simulink model "rah"  (Simulink 2.09)
settings: Solver=ode15s  StartTime=0.0  StopTime=60  MaxStep=5  RelTol=1e-6  AbsTol=1e-6
values from neighbouring files (symbols this model uses):
  dar = 0.165    [kpahrah.m]
  drr = -0.000075*Vref^2 + 0.0095*Vref - 0.4606    (= -0.184975)    [kpahrah.m]
  Ki_2 = 0.25    [kpahrah.m]
  Kphi = 0.000975*Vref^2 - 0.108*Vref + 2.335625    (= -0.55)    [kpahrah.m]
  Kr = -4    [kpahrah.m]
  refvelocity = 55    [actrload.m]    (also in prahinit.m = 45)
undefined symbols (not defined in the file or in its folder): Aail, AM, Arud, Bail, Brud, Cail, Crud, Dail, Drud, GM1, uaero0, uprop0, xfix, xinco
settings Model: SaveTime=off  SaveOutput=off  ConsistencyChecking=off  RTWTemplateMakefile=grt_vc.tmf

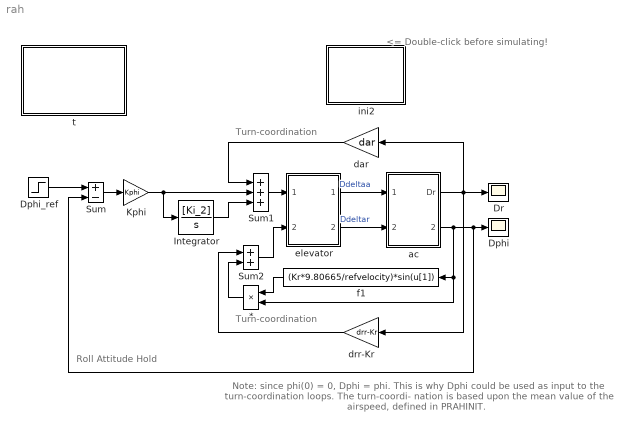
== system rah ==
  note: <= Double-click
      | before
      |   simulating!
  note: Note: since phi(0) = 0, Dphi = phi. This
      | is why Dphi could be used as input to the
      | turn-coordination loops. The turn-coordi-
      | nation is based upon the mean value of
      | the airspeed, defined in PRAHINIT.
  note: Roll Attitude Hold
  note: Turn-coordination
  note: Turn-coordination
  * : Product  Orientation=left  Inputs=2
  Dphi : Scope
      settings: TickLabels=on  TimeRange=60.000000  YMin=-0.300000  YMax=0.300000  SaveToWorkspace=off  SaveName=ScopeData
  Dphi_ref : Step  Time=0  Before=0  After=10*pi/180
  Dr : Scope
      settings: TickLabels=on  TimeRange=60.000000  YMin=-0.025000  YMax=0.025000  SaveToWorkspace=off  SaveName=ScopeData
  Integrator : TransferFcn  Numerator=[Ki_2]  Denominator=[1 0]
  Kphi : Gain  Gain=Kphi
  Sum : Sum  Inputs=+-
  Sum1 : Sum  Inputs=+++
  Sum2 : Sum  Inputs=++
  ac : Subsystem
      mask Display: disp('BEAVER\ndynamics')
  dar : Gain  Orientation=left  Gain=dar
  drr-Kr : Gain  Orientation=left  Gain=drr-Kr
  elevator : Subsystem
      mask Display: disp('Cable &\nactuator\ndynamics')
  f1 : Fcn  Orientation=left  Expr=(Kr*9.80665/refvelocity)*sin(u[1])
  ini2 : Subsystem
      settings: OpenFcn=prahinit
      mask Display: disp('Initialize\nmodel\n\nPRAHINIT')
  t : Subsystem
      mask Display: disp('RAH with\nturn-coordination\nwithout limiters.\nMarc Rauw,\nOctober 1997')
  wires:
  Dphi_ref/1 -> Sum/1
  Sum/1 -> Kphi/1
  elevator/1(Ddeltaa) -> ac/1(Ddelta_a)  "Ddeltaa"
  elevator/2(Ddeltar) -> ac/2(Ddelta_r)  "Ddeltar"
  Sum1/1 -> elevator/1(VDdeltaa)
  ac/1(Dr) -> Dr/1, dar/1, drr-Kr/1
  f1/1 -> */1
  Sum2/1 -> elevator/2(VDdeltar)
  */1 -> Sum2/2
  drr-Kr/1 -> Sum2/1
  ac/2(Dphi) -> f1/1, */2, Sum/2, Dphi/1
  Kphi/1 -> Sum1/2, Integrator/1
  Integrator/1 -> Sum1/3
  dar/1 -> Sum1/1

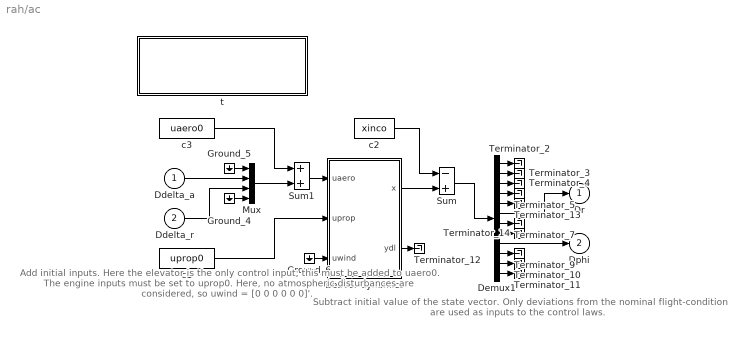
== system rah/ac ==
  note: Subtract initial value of  the state
      | vector. Only deviations from the
      | nominal flight-condition are used
      | as inputs to the control laws.
  note: Add initial inputs. Here the elevator
      | is the only control input; this must
      | be added to uaero0. The engine
      | inputs must be set to uprop0. Here,
      | no atmospheric disturbances are
      | considered, so uwind = [0 0 0 0 0 0]'.
  Ddelta_a : Inport  Port=1  PortWidth=-1  SampleTime=-1
  Ddelta_r : Inport  Port=2  PortWidth=-1  SampleTime=-1
  Beaver dynamics : Subsystem
  Demux1 : Demux  Outputs=12
  Ground_4 : Ground
  Ground_5 : Ground
  Ground_6 : Ground
  Mux : Mux  Inputs=4
  Sum : Sum  Inputs=-+
  Sum1 : Sum  Inputs=++
  Terminator_{2..5,7,9..14} (11 alike) : Terminator
  c1 : Constant  Value=uprop0
  c2 : Constant  Value=xinco
  c3 : Constant  Value=uaero0
  t : Subsystem
      mask Display: disp('Call subsystem-equivalent of the\nsystem BEAVER and convert\nI/O signals to small-deviations.\nMarc Rauw, October 1997')
  Dr : Outport  Port=1  InitialOutput=0
  Dphi : Outport  Port=2  InitialOutput=0
  wires:
  c3/1 -> Sum1/1
  c1/1 -> Beaver dynamics/2(uprop)
  c2/1 -> Sum/1
  Beaver dynamics/2(ydl) -> Terminator_12/1
  Beaver dynamics/1(x) -> Sum/2
  Demux1/1 -> Terminator_2/1
  Demux1/2 -> Terminator_3/1
  Demux1/3 -> Terminator_4/1
  Demux1/4 -> Terminator_5/1
  Demux1/7 -> Terminator_7/1
  Demux1/10 -> Terminator_9/1
  Demux1/11 -> Terminator_10/1
  Demux1/12 -> Terminator_11/1
  Sum/1 -> Demux1/1
  Sum1/1 -> Beaver dynamics/1(uaero)
  Mux/1 -> Sum1/2
  Ddelta_a/1 -> Mux/2
  Ground_5/1 -> Mux/1
  Ddelta_r/1 -> Mux/3
  Ground_4/1 -> Mux/4
  Ground_6/1 -> Beaver dynamics/3(uwind)
  Demux1/5 -> Terminator_13/1
  Demux1/8 -> Terminator_14/1
  Demux1/6 -> Dr/1
  Demux1/9 -> Dphi/1

== system rah/elevator ==
  note: Second inputs of Mux blocks take into account
      | influence of roll and yaw-rate upon aileron deflection
      | and rudder deflection, respectively (neglected here).
  VDdeltaa : Inport  Port=1  PortWidth=-1  SampleTime=-1
  VDdeltar : Inport  Port=2  PortWidth=-1  SampleTime=-1
  Ailerons actuator and cables : StateSpace  A=Aail  B=Bail  C=Cail  D=Dail  X0=0
  Ground_1 : Ground
  Ground_2 : Ground
  Mux : Mux  Inputs=2
  Mux1 : Mux  Inputs=2
  Rudder actuator and cables : StateSpace  A=Arud  B=Brud  C=Crud  D=Drud  X0=0
  t : Subsystem
      mask Display: disp('Dynamics of ailerons and\nrudder actuators and cables.\nMarc Rauw, October 1997')
  Ddeltaa : Outport  Port=1  InitialOutput=0
  Ddeltar : Outport  Port=2  InitialOutput=0
  wires:
  Ailerons actuator and cables/1 -> Ddeltaa/1
  VDdeltaa/1 -> Mux/1
  Mux/1 -> Ailerons actuator and cables/1
  Mux1/1 -> Rudder actuator and cables/1
  VDdeltar/1 -> Mux1/1
  Rudder actuator and cables/1 -> Ddeltar/1
  Ground_1/1 -> Mux/2
  Ground_2/1 -> Mux1/2

== system rah/ini2 ==

== system rah/t ==

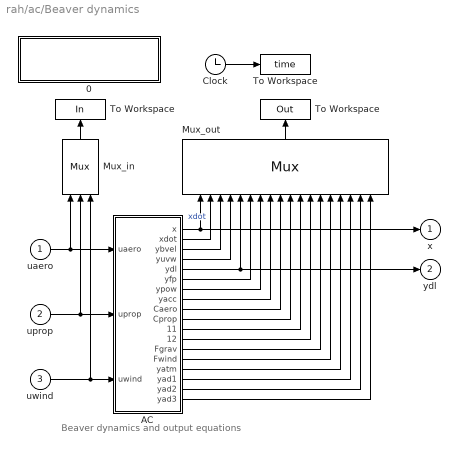
== system rah/ac/Beaver dynamics ==
  note: Beaver dynamics
      | and output equations
  uaero : Inport  Port=1  PortWidth=4  SampleTime=-1
  uprop : Inport  Port=2  PortWidth=2  SampleTime=-1
  uwind : Inport  Port=3  PortWidth=6  SampleTime=-1
  0 : Subsystem
      settings: OpenFcn=fdchelp level1
      mask Display: disp('Subsystem equivalent of\nthe S-function BEAVER\nM.O. Rauw, October 1997')
  AC : Subsystem
  Clock : Clock
  Mux_in : Mux  Orientation=up  Inputs=[4 2 6]
      settings: OpenFcn=fdchelp inputs
      mask Display: disp('Mux\nclick\n2x for\ninfo!')
  Mux_out : Mux  Orientation=up  Inputs=[12 12 3 3 3 4 2 6 6 6 6 6 3 3 5 3 3 3]
      settings: OpenFcn=fdchelp outputs
      mask Display: disp('Mux\n\nDouble-click for info!')
  To Workspace : ToWorkspace  VariableName=Out  SampleTime=0
      settings: Orientation=up  Buffer=5000
  "To Workspace " : ToWorkspace  VariableName=In  SampleTime=0
      settings: Orientation=up  Buffer=5000
  "To Workspace  " : ToWorkspace  VariableName=time  SampleTime=0
      settings: Buffer=5000
  x : Outport  Port=1  InitialOutput=0
  ydl : Outport  Port=2  InitialOutput=0
  wires:
  AC/7(ypow) -> Mux_out/7
  Mux_in/1 -> "To Workspace "/1
  Mux_out/1 -> To Workspace/1
  Clock/1 -> "To Workspace  "/1
  AC/15(yatm) -> Mux_out/15
  AC/14(Fwind) -> Mux_out/14
  AC/13(Fgrav) -> Mux_out/13
  AC/12(FMprop) -> Mux_out/12
  AC/11(FMaero) -> Mux_out/11
  AC/10(Cprop) -> Mux_out/10
  AC/9(Caero) -> Mux_out/9
  AC/8(yacc) -> Mux_out/8
  AC/6(yfp) -> Mux_out/6
  AC/5(ydl) -> ydl/1, Mux_out/5
  AC/16(yad1) -> Mux_out/16
  AC/3(ybvel) -> Mux_out/3
  AC/1(x) -> Mux_out/1, x/1
  AC/4(yuvw) -> Mux_out/4
  AC/17(yad2) -> Mux_out/17
  AC/18(yad3) -> Mux_out/18
  uwind/1 -> AC/3(" uwind"), Mux_in/3
  uprop/1 -> AC/2(uprop), Mux_in/2
  uaero/1 -> AC/1(uaero), Mux_in/1
  AC/2(xdot) -> Mux_out/2  "xdot"

== system rah/ac/t ==

== system rah/elevator/t ==

== system rah/ac/Beaver dynamics/0 ==

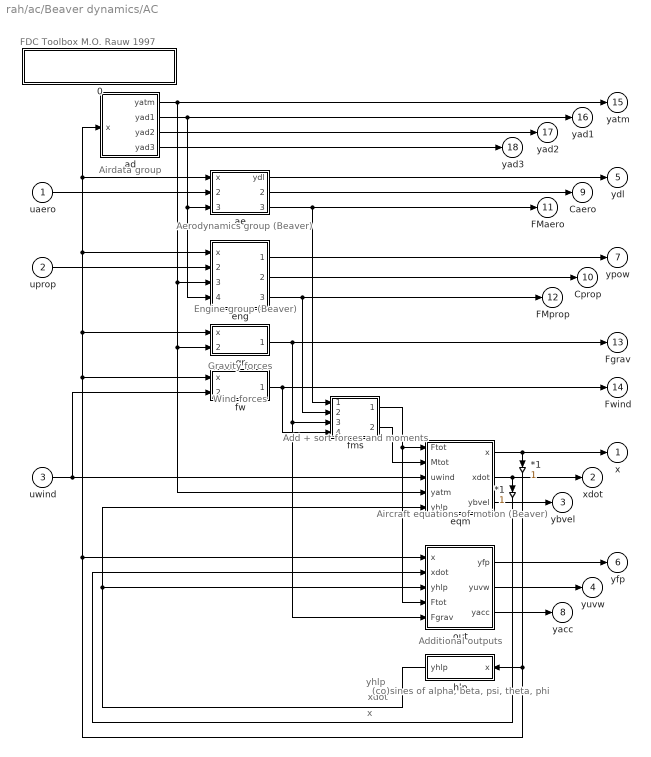
== system rah/ac/Beaver dynamics/AC ==
  note: FDC Toolbox
      |  M.O. Rauw 1997
  note: xdot
  note: x
  note: yhlp
  note: Additional outputs
  note: Aircraft equations
      | of motion (Beaver)
  note: Wind forces
  note: Gravity forces
  note: Engine group (Beaver)
  note: Aerodynamics
      | group (Beaver)
  note: (co)sines of
      | alpha, beta,
      | psi, theta, phi
  note: Add + sort
      | forces and
      | moments
  note: Airdata group
  uaero : Inport  Port=1  PortWidth=-1  SampleTime=-1
  uprop : Inport  Port=2  PortWidth=-1  SampleTime=-1
  " uwind" : Inport  Port=3  PortWidth=-1  SampleTime=-1
  " *1" : Gain  Orientation=down  Gain=1
  *1 : Gain  Orientation=down  Gain=1
  0 : Subsystem
      settings: OpenFcn=fdchelp level2
      mask Display: disp('BEAVER, level 2 (main level)\nM.O. Rauw')
  ad : Subsystem
  ae : Subsystem
  eng : Subsystem
  eqm : Subsystem
  fms : Subsystem
      mask Type: FMsort
      mask Description: Forces and Moments sorting block
      mask Help: eval('fdchelp fmsort')
      mask Display: disp('FMsort')
  fw : Subsystem  mask(fwind){m=GM1(10)}
      mask prompts: m "Mass of the aircraft [kg]:"
      mask help: Forces due to non-steady atmosphere.
      mask Help: eval('fdchelp fwind')
      mask Display: disp('Fwind')
  gr : Subsystem  mask(Gravity){m=GM1(10)}
      mask prompts: m "Mass of the aircraft [kg]:"
      mask help: Gravity forces.
      mask Help: eval('fdchelp gravity')
      mask Display: disp('Gravity')
  hlp : Subsystem  Orientation=left
      mask Type: Hlpfcn
      mask Description: Help sines and cosines
      mask Help: eval('fdchelp hlpfcn')
      mask Display: disp('hlpfcn')
  out : Subsystem
  x : Outport  Port=1  InitialOutput=0
  xdot : Outport  Port=2  InitialOutput=0
  ybvel : Outport  Port=3  InitialOutput=0
  yuvw : Outport  Port=4  InitialOutput=0
  ydl : Outport  Port=5  InitialOutput=0
  yfp : Outport  Port=6  InitialOutput=0
  ypow : Outport  Port=7  InitialOutput=0
  yacc : Outport  Port=8  InitialOutput=0
  Caero : Outport  Port=9  InitialOutput=0
  Cprop : Outport  Port=10  InitialOutput=0
  FMaero : Outport  Port=11  InitialOutput=0
  FMprop : Outport  Port=12  InitialOutput=0
  Fgrav : Outport  Port=13  InitialOutput=0
  Fwind : Outport  Port=14  InitialOutput=0
  yatm : Outport  Port=15  InitialOutput=0
  yad1 : Outport  Port=16  InitialOutput=0
  yad2 : Outport  Port=17  InitialOutput=0
  yad3 : Outport  Port=18  InitialOutput=0
  wires:
  out/2(yuvw) -> yuvw/1
  uprop/1 -> eng/2(uprop)
  uaero/1 -> ae/2(uaero)
  ad/4(yad3) -> yad3/1
  ae/1(ydl) -> ydl/1
  ae/2(Caero) -> Caero/1
  eng/1(ypow) -> ypow/1
  eng/2(Cprop) -> Cprop/1
  eqm/3(ybvel) -> ybvel/1
  out/1(yfp) -> yfp/1
  ad/2(yad1) -> eng/4(yad1), ae/3(yad1), yad1/1
  ad/3(yad2) -> yad2/1
  ad/1(yatm) -> yatm/1, eng/3(yatm), eqm/4(yatm), gr/2(yatm)
  out/3(yacc) -> yacc/1
  fw/1(Fwind) -> Fwind/1, fms/4(Fwind)
  eng/3(FMprop) -> FMprop/1, fms/2(FMprop)
  ae/3(FMaero) -> FMaero/1, fms/1(FMaero)
  hlp/1(yhlp) -> eqm/5(yhlp), out/3(yhlp)
  " uwind"/1 -> eqm/3(uwind), fw/2(uwind)
  *1/1 -> out/2(xdot)
  gr/1(Fgrav) -> Fgrav/1, fms/3(Fgrav), out/5(Fgrav)
  " *1"/1 -> hlp/1(x), out/1(x), fw/1(x), gr/1(x), eng/1(x), ae/1(x), ad/1(x)
  eqm/2(xdot) -> xdot/1, *1/1
  eqm/1(x) -> x/1, " *1"/1
  fms/1(Ftot) -> out/4(Ftot), eqm/1(Ftot)
  fms/2(Mtot) -> eqm/2(Mtot)

== system rah/ac/Beaver dynamics/AC/0 ==

== system rah/ac/Beaver dynamics/AC/ad ==
  x : Inport  Port=1  PortWidth=-1  SampleTime=-1
  0 : Subsystem
      settings: OpenFcn=fdchelp adgrp
      mask Display: disp('AIRDATA GROUP (level 3)\nM.O. Rauw')
  ad1 : Subsystem
      mask Type: Airdata1
      mask Description: Basic airdata variables
      mask Help: eval('fdchelp airdata1')
      mask Display: disp('Airdata1')
  ad2 : Subsystem
      mask Type: Airdata2
      mask Description: More airdata variables
      mask Help: eval('fdchelp airdata2')
      mask Display: disp('Airdata2')
  ad3 : Subsystem  mask(Airdata3){cbar=GM1(1)}
      mask prompts: cbar "Mean aerodynamic chord [m]:"
      mask help: More airdata variables
      mask Help: eval('fdchelp airdata3')
      mask Display: disp('Airdata3')
  atm : Subsystem
      mask Type: Atmosph
      mask Description: Atmosphere variables
      mask Help: eval('fdchelp atmosph')
      mask Display: disp('Atmosph')
  yatm : Outport  Port=1  InitialOutput=0
  yad1 : Outport  Port=2  InitialOutput=0
  yad2 : Outport  Port=3  InitialOutput=0
  yad3 : Outport  Port=4  InitialOutput=0
  wires:
  ad2/1(yad2) -> yad2/1
  ad3/1(yad3) -> yad3/1
  x/1 -> atm/1(x), ad1/1(x), ad3/1(x)
  atm/1(yatm) -> yatm/1, ad1/2(yatm), ad2/1(yatm), ad3/2(yatm)
  ad1/1(yad1) -> yad1/1, ad2/2(yad1), ad3/3(yad1)

== system rah/ac/Beaver dynamics/AC/ae ==
  x : Inport  Port=1  PortWidth=-1  SampleTime=-1
  uaero : Inport  Port=2  PortWidth=-1  SampleTime=-1
  yad1 : Inport  Port=3  PortWidth=-1  SampleTime=-1
  0 : Subsystem
      settings: OpenFcn=fdchelp aerogrp
      mask Display: disp('AERODYNAMICS GROUP (level 3)\nM.O. Rauw')
  aero : Subsystem
      mask Type: Aeromod
      mask Description: Aerodynamic model of the DHC-2 'Beaver'.
      mask Help: eval('fdchelp aeromod')
      mask Display: disp('Aeromod\n(Beaver)')
  dl : Subsystem  mask(Dimless){cbar=GM1(1), b=GM1(2)}
      mask prompts: cbar "Mean aerodynamic chord [m]:"; b "Wing span [m]:"
      mask help: Dimensionless rotational velocities.
      mask Help: eval('fdchelp dimless')
      mask Display: disp('Dimless')
  fmdims : Subsystem  mask(FMdims){cbar=GM1(1), b=GM1(2), S=GM1(3)}
      mask prompts: cbar "Mean aerodynamic chord [m]:"; b "Wing span [m]:"; S "Wing surface [m^2]:"
      mask help:
      | Calculate forces and moments from
      | dimensionless coefficients.
      mask Help: eval('fdchelp fmdims')
      mask Display: disp('FMdims')
  ydl : Outport  Port=1  InitialOutput=0
  Caero : Outport  Port=2  InitialOutput=0
  FMaero : Outport  Port=3  InitialOutput=0
  wires:
  aero/1(Caero) -> Caero/1, fmdims/2(Force / moment coefficients)
  dl/1(ydl) -> ydl/1, aero/3(ydl)
  x/1 -> dl/1(x), aero/1(x)
  uaero/1 -> aero/2(uaero)
  yad1/1 -> fmdims/1(yad1)
  fmdims/1(Forces and moments) -> FMaero/1

== system rah/ac/Beaver dynamics/AC/eng ==
  x : Inport  Port=1  PortWidth=-1  SampleTime=-1
  uprop : Inport  Port=2  PortWidth=-1  SampleTime=-1
  yatm : Inport  Port=3  PortWidth=-1  SampleTime=-1
  yad1 : Inport  Port=4  PortWidth=-1  SampleTime=-1
  0 : Subsystem
      settings: OpenFcn=fdchelp enggrp
      mask Display: disp('ENGINE GROUP (level 3)\nM.O. Rauw')
  eng : Subsystem
      mask Type: Engmod
      mask Description: Engine model for the DHC-2 'Beaver'
      mask Help: eval('fdchelp engmod')
      mask Display: disp('Engmod\n(Beaver)')
  fmdims : Subsystem  mask(FMdims){cbar=GM1(1), b=GM1(2), S=GM1(3)}
      mask prompts: cbar "Mean aerodynamic chord [m]:"; b "Wing span [m]:"; S "Wing surface [m^2]:"
      mask help:
      | Calculate forces and moments from
      | dimensionless coefficients.
      mask Help: eval('fdchelp fmdims')
      mask Display: disp('FMdims')
  pow : Subsystem
      mask Type: Power
      mask Description:
      | Engine power and dimensionless
      | pressure increase across propeller
      | (model for DHC-2 'Beaver')
      mask Help: eval('fdchelp power')
      mask Display: disp('Power\n(Beaver)')
  ypow : Outport  Port=1  InitialOutput=0
  Cprop : Outport  Port=2  InitialOutput=0
  FMprop : Outport  Port=3  InitialOutput=0
  wires:
  pow/1(ypow) -> ypow/1, eng/2(ypow)
  uprop/1 -> pow/2(uprop)
  fmdims/1(Forces and moments) -> FMprop/1
  eng/1(Cprop) -> Cprop/1, fmdims/2(Force / moment coefficients)
  yad1/1 -> fmdims/1(yad1)
  x/1 -> pow/1(x), eng/1(x)
  yatm/1 -> pow/3(yatm)

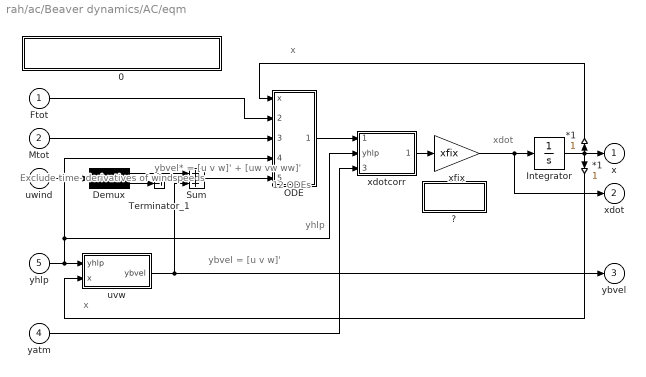
== system rah/ac/Beaver dynamics/AC/eqm ==
  note: Exclude time-
      | derivatives
      | of windspeeds
  note: ybvel* =
      | [u v w]' +
      | [uw vw ww]'
  note: xdot
  note: x
  note: x
  note: yhlp
  note: ybvel = [u v w]'
  note: 12 ODEs
  Ftot : Inport  Port=1  PortWidth=-1  SampleTime=-1
  Mtot : Inport  Port=2  PortWidth=-1  SampleTime=-1
  uwind : Inport  Port=3  PortWidth=-1  SampleTime=-1
  yatm : Inport  Port=4  PortWidth=-1  SampleTime=-1
  yhlp : Inport  Port=5  PortWidth=-1  SampleTime=-1
  " *1" : Gain  Orientation=up  Gain=1
  *1 : Gain  Orientation=down  Gain=1
  0 : Subsystem
      settings: OpenFcn=fdchelp eqmotion
      mask Display: disp('EQUATIONS OF MOTION (level 3)\nM.O. Rauw')
  "?" : Subsystem
      settings: OpenFcn=fdchelp xfix
      mask Display: disp('More info\nfor xfix')
  Demux : Demux  Outputs=[3 3]
  Integrator : Integrator  ExternalReset=none  InitialConditionSource=internal  InitialCondition=xinco  LimitOutput=off  UpperSaturationLimit=inf  LowerSaturationLimit=-inf  ShowSaturationPort=off  ShowStatePort=off  AbsoluteTolerance=auto
  ODE : Subsystem
  Sum : Sum  Inputs=++
  Terminator_1 : Terminator
  uvw : Subsystem
      mask Type: uvw
      mask Description:
      | Calculation of body-axes velocities
      | u, v, and w
      mask Help: eval('fdchelp uvw')
      mask Display: disp('Body-axes\nvelocities')
  xdotcorr : Subsystem  mask(xdotcorr){b=GM1(2), S=GM1(3), m=GM1(10), CYbdot=AM(2,19)}
      mask prompts: b "Wing span [m]:"; S "Wing surface [m^2]:"; m "Mass of the aircraft [kg]:"; CYbdot "Stability-derivative CYbdot:"
      mask help:
      | Correction block to write state
      | equations for DHC-2 Beaver aircraft
      | explicitly.
      mask Help: eval('fdchelp xdotcorr')
      mask Display: disp('xdotcorr\n(Beaver)')
  xfix : Gain  Gain=xfix
  x : Outport  Port=1  InitialOutput=0
  xdot : Outport  Port=2  InitialOutput=0
  ybvel : Outport  Port=3  InitialOutput=0
  wires:
  Demux/2 -> Terminator_1/1
  yhlp/1 -> uvw/1(yhlp), ODE/4(yhlp), xdotcorr/2(yhlp)
  ODE/1(xdot) -> xdotcorr/1(xdot uncorrected)
  Sum/1 -> ODE/5(ybvel*)
  uvw/1(ybvel) -> ybvel/1, Sum/2
  uwind/1 -> Demux/1
  Demux/1 -> Sum/1
  xdotcorr/1(xdot corrected) -> xfix/1
  yatm/1 -> xdotcorr/3(yatm)
  Ftot/1 -> ODE/2(Ftot)
  Mtot/1 -> ODE/3(Mtot)
  *1/1 -> uvw/2(x)
  Integrator/1 -> x/1, " *1"/1, *1/1
  xfix/1 -> Integrator/1, xdot/1
  " *1"/1 -> ODE/1(x)

== system rah/ac/Beaver dynamics/AC/fms ==
  note: `
  FMaero : Inport  Port=1  PortWidth=-1  SampleTime=-1
  FMprop : Inport  Port=2  PortWidth=-1  SampleTime=-1
  Fgrav : Inport  Port=3  PortWidth=-1  SampleTime=-1
  Fwind : Inport  Port=4  PortWidth=-1  SampleTime=-1
  0 : Subsystem
      settings: OpenFcn=fdchelp fmsort
      mask Display: disp('FMSORT\nM.O. Rauw, October 1997')
  Demux : Demux  Outputs=[3 3]
  Demux1 : Demux  Outputs=[3 3]
  Sum1 : Sum  Inputs=++
  Sum3 : Sum  Inputs=++++
  Ftot : Outport  Port=1  InitialOutput=0
  Mtot : Outport  Port=2  InitialOutput=0
  wires:
  FMaero/1 -> Demux/1
  FMprop/1 -> Demux1/1
  Demux1/2 -> Sum1/2
  Demux/2 -> Sum1/1
  Fgrav/1 -> Sum3/3
  Demux1/1 -> Sum3/2
  Sum3/1 -> Ftot/1
  Sum1/1 -> Mtot/1
  Demux/1 -> Sum3/1
  Fwind/1 -> Sum3/4

== system rah/ac/Beaver dynamics/AC/fw ==
  x : Inport  Port=1  PortWidth=-1  SampleTime=-1
  uwind : Inport  Port=2  PortWidth=-1  SampleTime=-1
  -Xw/m : Fcn  Expr=u[16] + u[5]*u[15] - u[6]*u[14]
  -Yw/m : Fcn  Expr=u[17] - u[4]*u[15] + u[6]*u[13]
  -Zw/m : Fcn  Expr=u[18] + u[4]*u[14] - u[5]*u[13]
  0 : Subsystem
      settings: OpenFcn=fdchelp fwind
      mask Display: disp('FWIND\nM.O. Rauw, Dec. 1996')
  Mux : Mux  Inputs=3
  Mux1 : Mux  Inputs=[12 6]
  gain : Gain  Gain=-m
  Fwind : Outport  Port=1  InitialOutput=0
  wires:
  uwind/1 -> Mux1/2
  x/1 -> Mux1/1
  gain/1 -> Fwind/1
  Mux/1 -> gain/1
  Mux1/1 -> -Yw/m/1, -Zw/m/1, -Xw/m/1
  -Yw/m/1 -> Mux/2
  -Xw/m/1 -> Mux/1
  -Zw/m/1 -> Mux/3

== system rah/ac/Beaver dynamics/AC/gr ==
  x : Inport  Port=1  PortWidth=-1  SampleTime=-1
  yatm : Inport  Port=2  PortWidth=-1  SampleTime=-1
  0 : Subsystem
      settings: OpenFcn=fdchelp gravity
      mask Display: disp('GRAVITY\nM.O. Rauw, October 1997')
  Mux : Mux  Inputs=3
  Mux1 : Mux  Inputs=[12 5]
  Xgr : Fcn  Expr=-m*u[17]*sin(u[8])
  Ygr : Fcn  Expr=m*u[17]*cos(u[8])*sin(u[9])
  Zgr : Fcn  Expr=m*u[17]*cos(u[8])*cos(u[9])
  Fgrav : Outport  Port=1  InitialOutput=0
  wires:
  Xgr/1 -> Mux/1
  Ygr/1 -> Mux/2
  Mux/1 -> Fgrav/1
  Mux1/1 -> Ygr/1, Xgr/1, Zgr/1
  Zgr/1 -> Mux/3
  x/1 -> Mux1/1
  yatm/1 -> Mux1/2

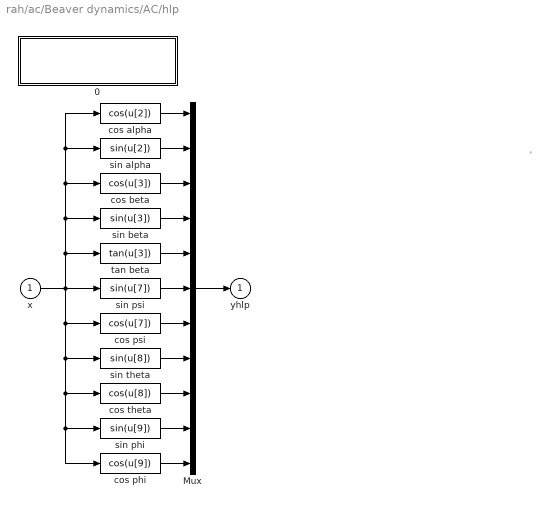
== system rah/ac/Beaver dynamics/AC/hlp ==
  note: '
  x : Inport  Port=1  PortWidth=-1  SampleTime=-1
  0 : Subsystem
      settings: OpenFcn=fdchelp hlpfcn
      mask Display: disp('HELP FUNCTIONS\n(often used sines and cosines)\nM.O. Rauw, October 1997')
  Mux : Mux  Inputs=11
  cos alpha : Fcn  Expr=cos(u[2])
  cos beta : Fcn  Expr=cos(u[3])
  cos phi : Fcn  Expr=cos(u[9])
  cos psi : Fcn  Expr=cos(u[7])
  cos theta : Fcn  Expr=cos(u[8])
  sin alpha : Fcn  Expr=sin(u[2])
  sin beta : Fcn  Expr=sin(u[3])
  sin phi : Fcn  Expr=sin(u[9])
  sin psi : Fcn  Expr=sin(u[7])
  sin theta : Fcn  Expr=sin(u[8])
  tan beta : Fcn  Expr=tan(u[3])
  yhlp : Outport  Port=1  InitialOutput=0
  wires:
  x/1 -> sin psi/1, sin beta/1, cos beta/1, sin alpha/1, cos alpha/1, tan beta/1, sin theta/1, cos theta/1, sin phi/1, cos phi/1, cos psi/1
  cos alpha/1 -> Mux/1
  sin alpha/1 -> Mux/2
  cos beta/1 -> Mux/3
  sin beta/1 -> Mux/4
  tan beta/1 -> Mux/5
  sin psi/1 -> Mux/6
  cos psi/1 -> Mux/7
  sin theta/1 -> Mux/8
  cos theta/1 -> Mux/9
  sin phi/1 -> Mux/10
  Mux/1 -> yhlp/1
  cos phi/1 -> Mux/11

== system rah/ac/Beaver dynamics/AC/out ==
  note: Flightpath
      | variables
  note: du/dt, dv/dt, dw/dt
      | (output equations!)
  note: Body-axes accelerations
      | and specific forces
  x : Inport  Port=1  PortWidth=-1  SampleTime=-1
  xdot : Inport  Port=2  PortWidth=-1  SampleTime=-1
  yhlp : Inport  Port=3  PortWidth=-1  SampleTime=-1
  Ftot : Inport  Port=4  PortWidth=-1  SampleTime=-1
  Fgrav : Inport  Port=5  PortWidth=-1  SampleTime=-1
  0 : Subsystem
      settings: OpenFcn=fdchelp moreouts
      mask Display: disp('Additional outputs (level 3)\nM.O. Rauw')
  accel : Subsystem  mask(accel){m=GM1(10)}
      mask prompts: m "Mass of the aircraft [kg]:"
      mask help:
      | Body axes accelerations and
      | specific forces.
      mask Help: eval('fdchelp accel')
      mask Display: disp('Accel')
  fp : Subsystem  mask(Flpath){alpha0=xinco(2)}
      mask prompts: alpha0 "Initial value of angle of attack, alpha0:"
      mask help: Flightpath related parameters.
      mask Help: eval('fdchelp flpath')
      mask Display: disp('flpath')
  uvwdot : Subsystem
      mask Type: uvwdot
      mask Description: Calculation of du/dt, dv/dt, and dw/dt.
      mask Help: eval('fdchelp uvwdot')
      mask Display: disp('uvwdot')
  yfp : Outport  Port=1  InitialOutput=0
  yuvw : Outport  Port=2  InitialOutput=0
  yacc : Outport  Port=3  InitialOutput=0
  wires:
  fp/1(yfp) -> yfp/1
  uvwdot/1(yuvw =  [udot; vdot; wdot]) -> yuvw/1
  yhlp/1 -> uvwdot/3(yhlp)
  Ftot/1 -> accel/1(Ftot)
  accel/1(yacc) -> yacc/1
  xdot/1 -> fp/2(xdot), uvwdot/2(xdot)
  x/1 -> fp/1(x), uvwdot/1(x)
  Fgrav/1 -> accel/2(Fgrav)

== system rah/ac/Beaver dynamics/AC/ad/0 ==

== system rah/ac/Beaver dynamics/AC/ad/ad1 ==
  x : Inport  Port=1  PortWidth=-1  SampleTime=-1
  yatm : Inport  Port=2  PortWidth=-1  SampleTime=-1
  0 : Subsystem
      settings: OpenFcn=fdchelp airdata1
      mask Display: disp('AIRDATA1\nM.O. Rauw, October 1997')
  M : Fcn  Expr=u[2]/u[1]
  Mux : Mux  Inputs=[1 12]
  Mux1 : Mux  Inputs=[12 5]
  Mux2 : Mux  Inputs=3
  a : Fcn  Expr=sqrt(401.8743*u[3])
  qdyn : Fcn  Expr=0.5*u[13]*u[1]^2
  yad1 : Outport  Port=1  InitialOutput=0
  wires:
  Mux2/1 -> yad1/1
  qdyn/1 -> Mux2/3
  a/1 -> Mux/1, Mux2/1
  M/1 -> Mux2/2
  Mux1/1 -> qdyn/1
  Mux/1 -> M/1
  x/1 -> Mux/2, Mux1/1
  yatm/1 -> a/1, Mux1/2

== system rah/ac/Beaver dynamics/AC/ad/ad2 ==
  yatm : Inport  Port=1  PortWidth=-1  SampleTime=-1
  yad1 : Inport  Port=2  PortWidth=-1  SampleTime=-1
  0 : Subsystem
      settings: OpenFcn=fdchelp airdata2
      mask Display: disp('AIRDATA2\nM.O. Rauw, October 1997')
  Mux : Mux  Inputs=[5 3]
  Mux1 : Mux  Inputs=3
  Vc : Fcn  Expr=sqrt(579000*((1+u[1]/101325)^(1/3.5)-1))
  Ve : Fcn  Expr=sqrt(u[8] * 1.63265)
  qc : Fcn  Expr=u[2] * ((1+0.2*u[7]^2)^3.5-1)
  yad2 : Outport  Port=1  InitialOutput=0
  wires:
  yad1/1 -> Mux/2
  yatm/1 -> Mux/1
  Mux/1 -> qc/1, Ve/1
  Ve/1 -> Mux1/2
  Vc/1 -> Mux1/3
  qc/1 -> Vc/1, Mux1/1
  Mux1/1 -> yad2/1

== system rah/ac/Beaver dynamics/AC/ad/ad3 ==
  x : Inport  Port=1  PortWidth=-1  SampleTime=-1
  yatm : Inport  Port=2  PortWidth=-1  SampleTime=-1
  yad1 : Inport  Port=3  PortWidth=-1  SampleTime=-1
  0 : Subsystem
      settings: OpenFcn=fdchelp airdata3
      mask Display: disp('AIRDATA3\nM.O. Rauw, October 1997')
  Mux : Mux  Inputs=3
  Mux1 : Mux  Inputs=[12 5 3]
  Re : Fcn  Expr=(u[13]*u[1])/u[16]
  Tt : Fcn  Expr=u[15] * (1+0.2*u[19]^2)
  cbar : Gain  Gain=cbar
  yad3 : Outport  Port=1  InitialOutput=0
  wires:
  yad1/1 -> Mux1/3
  yatm/1 -> Mux1/2
  x/1 -> Mux1/1
  Re/1 -> Mux/2, cbar/1
  Mux1/1 -> Re/1, Tt/1
  Mux/1 -> yad3/1
  Tt/1 -> Mux/1
  cbar/1 -> Mux/3

== system rah/ac/Beaver dynamics/AC/ad/atm ==
  x : Inport  Port=1  PortWidth=-1  SampleTime=-1
  0 : Subsystem
      settings: OpenFcn=fdchelp atmosph
      mask Display: disp('ATMOSPH\nM.O. Rauw, October 1997')
  Mux : Mux  Inputs=2
  Mux1 : Mux  Inputs=[2 1]
  Mux2 : Mux  Inputs=5
  T : Fcn  Expr=288.15 - 0.0065*u[12]
  g : Fcn  Expr=9.80665*(6371020/(6371020+u[12]))^2
  mu : Fcn  Expr=(1.458*10^(-6)*u[2]^1.5)/(u[2]+110.4)
  ps : Fcn  Expr=101325*(u[2]/288.15)^(u[1]/1.86584)
  rho : Fcn  Expr=u[3]/(287.053*u[2])
  yatm : Outport  Port=1  InitialOutput=0
  wires:
  x/1 -> T/1, g/1
  Mux/1 -> Mux1/1, mu/1, ps/1
  ps/1 -> Mux1/2, Mux2/2
  T/1 -> Mux/2, Mux2/3
  g/1 -> Mux/1, Mux2/5
  rho/1 -> Mux2/1
  Mux1/1 -> rho/1
  Mux2/1 -> yatm/1
  mu/1 -> Mux2/4

== system rah/ac/Beaver dynamics/AC/ae/0 ==

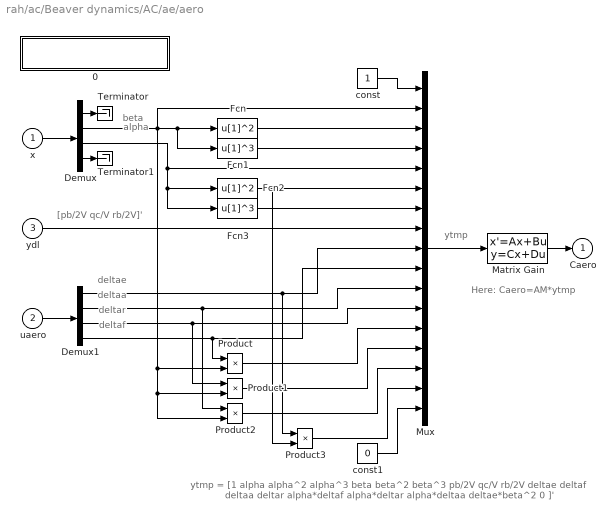
== system rah/ac/Beaver dynamics/AC/ae/aero ==
  note: ytmp = [1  alpha  alpha^2  alpha^3  beta  beta^2  beta^3  pb/2V  qc/V  rb/2V  deltae
      | deltaf  deltaa  deltar  alpha*deltaf  alpha*deltar  alpha*deltaa  deltae*beta^2  0 ]'
  note: [pb/2V qc/V rb/2V]'
  note: beta
  note: deltae
  note: deltaa
  note: deltar
  note: deltaf
  note: alpha
  note: ytmp
  note: Here: Caero=AM*ytmp
  x : Inport  Port=1  PortWidth=-1  SampleTime=-1
  uaero : Inport  Port=2  PortWidth=-1  SampleTime=-1
  ydl : Inport  Port=3  PortWidth=-1  SampleTime=-1
  0 : Subsystem
      settings: OpenFcn=fdchelp aeromod
      mask Display: disp('AEROMOD\nM.O. Rauw, October 1997')
  Demux : Demux  Outputs=[1 1 1 9]
  Demux1 : Demux  Outputs=4
  Fcn : Fcn  Expr=u[1]^2
  Fcn1 : Fcn  Expr=u[1]^3
  Fcn2 : Fcn  Expr=u[1]^2
  Fcn3 : Fcn  Expr=u[1]^3
  Matrix Gain : StateSpace  A=A  B=B  C=C  D=D  X0=0  mask(Matrix Gain){@1=AM}
      mask prompts: @1 "Gain matrix:"
      mask help: Matrix Gain
      mask init:
      | A = []; B = []; C = []; D = @1;
      mask Help: This block implements an matrix gain.\nThe matrix dimensions must be in accordance\nwith the dimension of the inputvector.
      mask Display: disp('y = A*u')
  Mux : Mux  Inputs=[1 1 1 1 1 1 1 3 1 1 1 1 1 1 1 1 1]
  Product{,1..3} (4 alike) : Product  Inputs=2
  Terminator : Terminator
  Terminator1 : Terminator
  const : Constant  Value=1
  const1 : Constant  Value=0
  Caero : Outport  Port=1  InitialOutput=0
  wires:
  Demux/4 -> Terminator1/1
  Demux/1 -> Terminator/1
  const1/1 -> Mux/17
  const/1 -> Mux/1
  ydl/1 -> Mux/8
  Product3/1 -> Mux/16
  Product2/1 -> Mux/15
  Product1/1 -> Mux/14
  Demux1/1 -> Mux/9, Product3/1
  Fcn2/1 -> Mux/6, Product3/2
  Demux1/4 -> Mux/10, Product/1
  Demux/2 -> Mux/2, Fcn/1, Fcn1/1, Product/2, Product1/2, Product2/2
  Demux/3 -> Mux/5, Fcn2/1, Fcn3/1
  Demux1/2 -> Mux/11, Product2/1
  Demux1/3 -> Mux/12, Product1/1
  Product/1 -> Mux/13
  Fcn3/1 -> Mux/7
  uaero/1 -> Demux1/1
  Fcn1/1 -> Mux/4
  Fcn/1 -> Mux/3
  x/1 -> Demux/1
  Mux/1 -> Matrix Gain/1
  Matrix Gain/1 -> Caero/1

== system rah/ac/Beaver dynamics/AC/ae/dl ==
  x : Inport  Port=1  PortWidth=-1  SampleTime=-1
  0 : Subsystem
      settings: OpenFcn=fdchelp dimless
      mask Display: disp('DIMLESS\nM.O. Rauw, October 1997')
  Mux : Mux  Inputs=3
  pb/2V : Fcn  Expr=0.5 * u[4] * b / u[1]
  qc/V : Fcn  Expr=u[5] * cbar / u[1]
  rb/2V : Fcn  Expr=0.5 * u[6] * b / u[1]
  ydl : Outport  Port=1  InitialOutput=0
  wires:
  pb/2V/1 -> Mux/1
  qc/V/1 -> Mux/2
  rb/2V/1 -> Mux/3
  Mux/1 -> ydl/1
  x/1 -> qc/V/1, rb/2V/1, pb/2V/1

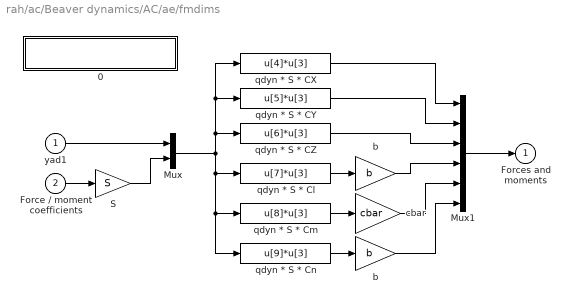
== system rah/ac/Beaver dynamics/AC/ae/fmdims ==
  yad1 : Inport  Port=1  PortWidth=-1  SampleTime=-1
  Force / moment coefficients : Inport  Port=2  PortWidth=-1  SampleTime=-1
  0 : Subsystem
      settings: OpenFcn=fdchelp fmdims
      mask Display: disp('FMDIMS\nM.O. Rauw, October 1997')
  Mux : Mux  Inputs=[3 6]
  Mux1 : Mux  Inputs=6
  S : Gain  Gain=S
  b : Gain  Gain=b
  "b " : Gain  Gain=b
  cbar : Gain  Gain=cbar
  qdyn * S * CX : Fcn  Expr=u[4]*u[3]
  qdyn * S * CY : Fcn  Expr=u[5]*u[3]
  qdyn * S * CZ : Fcn  Expr=u[6]*u[3]
  qdyn * S * Cl : Fcn  Expr=u[7]*u[3]
  qdyn * S * Cm : Fcn  Expr=u[8]*u[3]
  qdyn * S * Cn : Fcn  Expr=u[9]*u[3]
  Forces and moments : Outport  Port=1  InitialOutput=0
  wires:
  Mux1/1 -> Forces and moments/1
  "b "/1 -> Mux1/6
  cbar/1 -> Mux1/5
  Force / moment coefficients/1 -> S/1
  Mux/1 -> qdyn * S * CZ/1, qdyn * S * CX/1, qdyn * S * CY/1, qdyn * S * Cl/1, qdyn * S * Cm/1, qdyn * S * Cn/1
  qdyn * S * Cl/1 -> b/1
  qdyn * S * Cm/1 -> cbar/1
  qdyn * S * Cn/1 -> "b "/1
  yad1/1 -> Mux/1
  qdyn * S * CX/1 -> Mux1/1
  qdyn * S * CY/1 -> Mux1/2
  S/1 -> Mux/2
  qdyn * S * CZ/1 -> Mux1/3
  b/1 -> Mux1/4

== system rah/ac/Beaver dynamics/AC/eng/0 ==

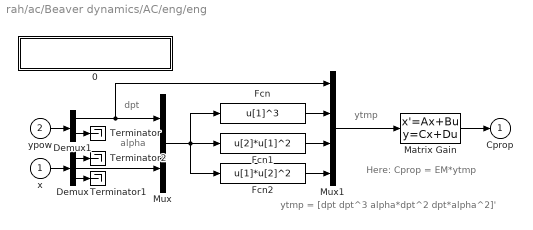
== system rah/ac/Beaver dynamics/AC/eng/eng ==
  note: Here: Cprop = EM*ytmp
  note: ytmp = [dpt dpt^3 alpha*dpt^2 dpt*alpha^2]'
  note: dpt
  note: alpha
  note: ytmp
  x : Inport  Port=1  PortWidth=-1  SampleTime=-1
  ypow : Inport  Port=2  PortWidth=-1  SampleTime=-1
  0 : Subsystem
      settings: OpenFcn=fdchelp engmod
      mask Display: disp('ENGMOD\nM.O. Rauw, Dec. 1996')
  Demux : Demux  Outputs=[1 1 10]
  Demux1 : Demux  Outputs=2
  Fcn : Fcn  Expr=u[1]^3
  Fcn1 : Fcn  Expr=u[2]*u[1]^2
  Fcn2 : Fcn  Expr=u[1]*u[2]^2
  Matrix Gain : StateSpace  A=A  B=B  C=C  D=D  X0=0  mask(Matrix Gain){@1=EM}
      mask prompts: @1 "Gain matrix:"
      mask help: Matrix Gain
      mask init:
      | A = []; B = []; C = []; D = @1;
      mask Help: This block implements an matrix gain.\nThe matrix dimensions must be in accordance\nwith the dimension of the inputvector.
      mask Display: disp('y = A*u')
  Mux : Mux  Inputs=2
  Mux1 : Mux  Inputs=4
  Terminator : Terminator
  Terminator1 : Terminator
  Terminator2 : Terminator
  Cprop : Outport  Port=1  InitialOutput=0
  wires:
  Demux/1 -> Terminator2/1
  Demux/3 -> Terminator1/1
  Demux1/2 -> Terminator/1
  Matrix Gain/1 -> Cprop/1
  Mux1/1 -> Matrix Gain/1
  x/1 -> Demux/1
  ypow/1 -> Demux1/1
  Demux/2 -> Mux/2
  Mux/1 -> Fcn1/1, Fcn/1, Fcn2/1
  Demux1/1 -> Mux/1, Mux1/1
  Fcn/1 -> Mux1/2
  Fcn1/1 -> Mux1/3
  Fcn2/1 -> Mux1/4

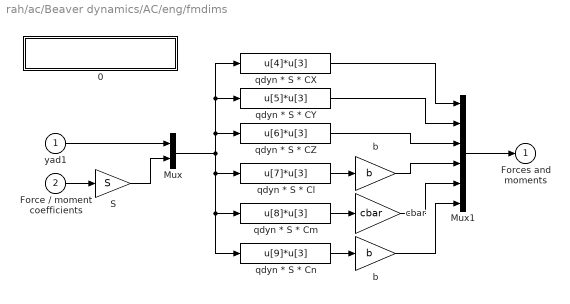
== system rah/ac/Beaver dynamics/AC/eng/fmdims ==
  yad1 : Inport  Port=1  PortWidth=-1  SampleTime=-1
  Force / moment coefficients : Inport  Port=2  PortWidth=-1  SampleTime=-1
  0 : Subsystem
      settings: OpenFcn=fdchelp fmdims
      mask Display: disp('FMDIMS\nM.O. Rauw, October 1997')
  Mux : Mux  Inputs=[3 6]
  Mux1 : Mux  Inputs=6
  S : Gain  Gain=S
  b : Gain  Gain=b
  "b " : Gain  Gain=b
  cbar : Gain  Gain=cbar
  qdyn * S * CX : Fcn  Expr=u[4]*u[3]
  qdyn * S * CY : Fcn  Expr=u[5]*u[3]
  qdyn * S * CZ : Fcn  Expr=u[6]*u[3]
  qdyn * S * Cl : Fcn  Expr=u[7]*u[3]
  qdyn * S * Cm : Fcn  Expr=u[8]*u[3]
  qdyn * S * Cn : Fcn  Expr=u[9]*u[3]
  Forces and moments : Outport  Port=1  InitialOutput=0
  wires:
  Mux1/1 -> Forces and moments/1
  "b "/1 -> Mux1/6
  cbar/1 -> Mux1/5
  Force / moment coefficients/1 -> S/1
  Mux/1 -> qdyn * S * CZ/1, qdyn * S * CX/1, qdyn * S * CY/1, qdyn * S * Cl/1, qdyn * S * Cm/1, qdyn * S * Cn/1
  qdyn * S * Cl/1 -> b/1
  qdyn * S * Cm/1 -> cbar/1
  qdyn * S * Cn/1 -> "b "/1
  yad1/1 -> Mux/1
  qdyn * S * CX/1 -> Mux1/1
  qdyn * S * CY/1 -> Mux1/2
  S/1 -> Mux/2
  qdyn * S * CZ/1 -> Mux1/3
  b/1 -> Mux1/4

== system rah/ac/Beaver dynamics/AC/eng/pow ==
  x : Inport  Port=1  PortWidth=-1  SampleTime=-1
  uprop : Inport  Port=2  PortWidth=-1  SampleTime=-1
  yatm : Inport  Port=3  PortWidth=-1  SampleTime=-1
  0 : Subsystem
      settings: OpenFcn=fdchelp power
      mask Display: disp('POWER\nM.O. Rauw, October 1997')
  Mux : Mux  Inputs=[12 2 5]
  Mux1 : Mux  Inputs=[19 1]
  Mux2 : Mux  Inputs=2
  P : Fcn  Expr=0.7355*(-326.5+0.00412*(u[14]+7.4)*(u[13]+2010)+(408.0-0.0965*u[13])*(1.0-u[15]/1.225))
  dpt : Fcn  Expr=0.08696 + 191.18*(u[20]/(0.5*u[15]*u[1]^3))
  ypow : Outport  Port=1  InitialOutput=0
  wires:
  Mux2/1 -> ypow/1
  dpt/1 -> Mux2/1
  yatm/1 -> Mux/3
  uprop/1 -> Mux/2
  x/1 -> Mux/1
  Mux/1 -> P/1, Mux1/1
  P/1 -> Mux2/2, Mux1/2
  Mux1/1 -> dpt/1

== system rah/ac/Beaver dynamics/AC/eqm/0 ==

== system rah/ac/Beaver dynamics/AC/eqm/? ==

== system rah/ac/Beaver dynamics/AC/eqm/ODE ==
  x : Inport  Port=1  PortWidth=-1  SampleTime=-1
  Ftot : Inport  Port=2  PortWidth=-1  SampleTime=-1
  Mtot : Inport  Port=3  PortWidth=-1  SampleTime=-1
  yhlp : Inport  Port=4  PortWidth=-1  SampleTime=-1
  ybvel* : Inport  Port=5  PortWidth=-1  SampleTime=-1
  0 : Subsystem
      settings: OpenFcn=fdchelp 12odes
      mask Display: disp('12 Ordinary Differential\nEquations (level 4)\nM.O. Rauw')
  Eulerdot : Subsystem
      mask Type: Eulerdot
      mask Description:
      | Calculation of d(psi)/dt, d(theta)/dt,
      | and d(phi/dt)
      mask Help: eval('fdchelp eulerdot')
      mask Display: disp('psi dot\ntheta dot\nphi dot')
  Mux : Mux  Inputs=[12 3 3 11]
  Mux1 : Mux  Inputs=[3 3 3 3]
  Vabdot : Subsystem  mask(Vabdot){m=GM1(10)}
      mask prompts: m "Mass of the aircraft [kg]:"
      mask help: Calculation of dV/dt, dalpha/dt, dbeta/dt.
      mask Help: eval('fdchelp vabdot')
      mask Display: disp('V dot\nalpha dot\nbeta dot')
  pqrdot : Subsystem
      mask Type: pqrdot
      mask Description: Calculation of dp/dt, dq/dt, and dr/dt
      mask Help: eval('fdchelp pqrdot')
      mask Display: disp('p dot\nq dot\nr dot')
  xyHdot : Subsystem
      mask Type: xyHdot
      mask Description: Calculation of d(xe)/dt, d(ye)/dt, and dH/dt
      mask Help: eval('fdchelp xyhdot')
      mask Display: disp('xe dot\nye dot\nH dot')
  xdot : Outport  Port=1  InitialOutput=0
  wires:
  x/1 -> Mux/1
  Mtot/1 -> Mux/3
  Ftot/1 -> Mux/2
  Mux/1 -> pqrdot/1(upqr), Vabdot/1(uVab), Eulerdot/1(ueul), xyHdot/2(uxYH)
  ybvel*/1 -> xyHdot/1(ybvel*)
  yhlp/1 -> Mux/4
  xyHdot/1(yxyH) -> Mux1/4
  Eulerdot/1(yeul) -> Mux1/3
  pqrdot/1(ypqr) -> Mux1/2
  Vabdot/1(yVab) -> Mux1/1
  Mux1/1 -> xdot/1

== system rah/ac/Beaver dynamics/AC/eqm/uvw ==
  yhlp : Inport  Port=1  PortWidth=-1  SampleTime=-1
  x : Inport  Port=2  PortWidth=-1  SampleTime=-1
  0 : Subsystem
      settings: OpenFcn=fdchelp uvw
      mask Display: disp('UVW\nM.O. Rauw, October 1997')
  Mux : Mux  Inputs=3
  Mux1 : Mux  Inputs=[12 11]
  u : Fcn  Expr=u[1]*u[13]*u[15]
  v : Fcn  Expr=u[1]*u[16]
  w : Fcn  Expr=u[1]*u[14]*u[15]
  ybvel : Outport  Port=1  InitialOutput=0
  wires:
  Mux1/1 -> v/1, u/1, w/1
  yhlp/1 -> Mux1/2
  x/1 -> Mux1/1
  u/1 -> Mux/1
  v/1 -> Mux/2
  w/1 -> Mux/3
  Mux/1 -> ybvel/1

== system rah/ac/Beaver dynamics/AC/eqm/xdotcorr ==
  xdot uncorrected : Inport  Port=1  PortWidth=-1  SampleTime=-1
  yhlp : Inport  Port=2  PortWidth=-1  SampleTime=-1
  yatm : Inport  Port=3  PortWidth=-1  SampleTime=-1
  0 : Subsystem
      settings: OpenFcn=fdchelp xdotcorr
      mask Display: disp('XDOTCORR (Beaver)\nM.O. Rauw, October 1997')
  Demux : Demux  Outputs=12
  Mux1 : Mux  Inputs=12
  Mux2 : Mux  Inputs=[11 1 5]
  beta dot correction : Fcn  Expr=u[12] / (1 - (u[3]*u[13]*b*S*CYbdot)/(4*m))
  xdot corrected : Outport  Port=1  InitialOutput=0
  wires:
  beta dot correction/1 -> Mux1/3
  yatm/1 -> Mux2/3
  Demux/1 -> Mux1/1
  Demux/2 -> Mux1/2
  Demux/4 -> Mux1/4
  Demux/5 -> Mux1/5
  Demux/6 -> Mux1/6
  Demux/7 -> Mux1/7
  Demux/8 -> Mux1/8
  Demux/9 -> Mux1/9
  Demux/10 -> Mux1/10
  Demux/11 -> Mux1/11
  Demux/12 -> Mux1/12
  Demux/3 -> Mux2/2
  xdot uncorrected/1 -> Demux/1
  Mux1/1 -> xdot corrected/1
  Mux2/1 -> beta dot correction/1
  yhlp/1 -> Mux2/1

== system rah/ac/Beaver dynamics/AC/fms/0 ==

== system rah/ac/Beaver dynamics/AC/fw/0 ==

== system rah/ac/Beaver dynamics/AC/gr/0 ==

== system rah/ac/Beaver dynamics/AC/hlp/0 ==

== system rah/ac/Beaver dynamics/AC/out/0 ==

== system rah/ac/Beaver dynamics/AC/out/accel ==
  Ftot : Inport  Port=1  PortWidth=-1  SampleTime=-1
  Fgrav : Inport  Port=2  PortWidth=-1  SampleTime=-1
  0 : Subsystem
      settings: OpenFcn=fdchelp accel
      mask Display: disp('ACCEL\nM.O. Rauw, October 1997')
  Ax : Fcn  Expr=(u[1]-u[4])/(m*9.80665)
  Ay : Fcn  Expr=(u[2]-u[5])/(m*9.80665)
  Az : Fcn  Expr=(u[3]-u[6])/(m*9.80665)
  Mux : Mux  Inputs=6
  Mux1 : Mux  Inputs=[3 3]
  axk : Fcn  Expr=u[1]/(m*9.80665)
  ayk : Fcn  Expr=u[2]/(m*9.80665)
  azk : Fcn  Expr=u[3]/(m*9.80665)
  yacc : Outport  Port=1  InitialOutput=0
  wires:
  Ftot/1 -> Mux1/1
  Fgrav/1 -> Mux1/2
  Mux/1 -> yacc/1
  azk/1 -> Mux/6
  Az/1 -> Mux/3
  Ay/1 -> Mux/2
  Ax/1 -> Mux/1
  Mux1/1 -> Az/1, Ax/1, Ay/1, axk/1, azk/1, ayk/1
  axk/1 -> Mux/4
  ayk/1 -> Mux/5

== system rah/ac/Beaver dynamics/AC/out/fp ==
  x : Inport  Port=1  PortWidth=-1  SampleTime=-1
  xdot : Inport  Port=2  PortWidth=-1  SampleTime=-1
  0 : Subsystem
      settings: OpenFcn=fdchelp flpath
      mask Display: disp('FLPATH\nM.O. Rauw, October 1997')
  Mux : Mux  Inputs=[12 12]
  Mux1 : Mux  Inputs=4
  Phi : Fcn  Expr=u[9]*cos(u[8]-alpha0)
  chi : Fcn  Expr=u[3]+u[7]
  fpa : Fcn  Expr=u[13]/9.80665
  gamma : Fcn  Expr=asin(u[24]/u[1])
  yfp : Outport  Port=1  InitialOutput=0
  wires:
  Mux/1 -> chi/1, Phi/1, fpa/1, gamma/1
  gamma/1 -> Mux1/1
  fpa/1 -> Mux1/2
  chi/1 -> Mux1/3
  Phi/1 -> Mux1/4
  Mux1/1 -> yfp/1
  x/1 -> Mux/1
  xdot/1 -> Mux/2

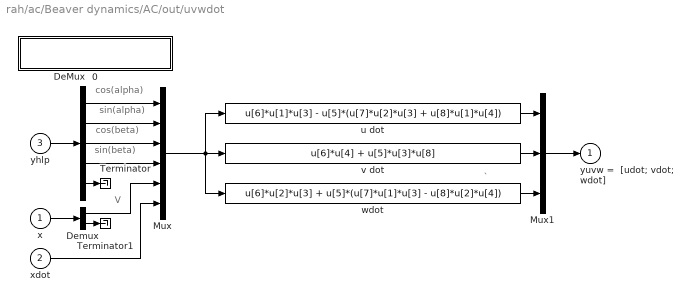
== system rah/ac/Beaver dynamics/AC/out/uvwdot ==
  note: `
  note: cos(alpha)
  note: sin(alpha)
  note: cos(beta)
  note: sin(beta)
  note: V
  x : Inport  Port=1  PortWidth=-1  SampleTime=-1
  xdot : Inport  Port=2  PortWidth=-1  SampleTime=-1
  yhlp : Inport  Port=3  PortWidth=-1  SampleTime=-1
  0 : Subsystem
      settings: OpenFcn=fdchelp uvwdot
      mask Display: disp('UVWDOT\nM.O. Rauw, October 1997')
  DeMux : Demux  Outputs=[1 1 1 1 7]
  Demux : Demux  Outputs=[1 11]
  Mux : Mux  Inputs=[1 1 1 1 1 12]
  Mux1 : Mux  Inputs=3
  Terminator : Terminator
  Terminator1 : Terminator
  u dot : Fcn  Expr=u[6]*u[1]*u[3] - u[5]*(u[7]*u[2]*u[3] + u[8]*u[1]*u[4])
  v dot : Fcn  Expr=u[6]*u[4] + u[5]*u[3]*u[8]
  wdot : Fcn  Expr=u[6]*u[2]*u[3] + u[5]*(u[7]*u[1]*u[3] - u[8]*u[2]*u[4])
  yuvw =  [udot; vdot; wdot] : Outport  Port=1  InitialOutput=0
  wires:
  Demux/2 -> Terminator1/1
  DeMux/5 -> Terminator/1
  wdot/1 -> Mux1/3
  v dot/1 -> Mux1/2
  u dot/1 -> Mux1/1
  xdot/1 -> Mux/6
  Mux/1 -> v dot/1, wdot/1, u dot/1
  DeMux/1 -> Mux/1
  DeMux/2 -> Mux/2
  x/1 -> Demux/1
  Mux1/1 -> yuvw =  [udot; vdot; wdot]/1
  yhlp/1 -> DeMux/1
  DeMux/3 -> Mux/3
  DeMux/4 -> Mux/4
  Demux/1 -> Mux/5

== system rah/ac/Beaver dynamics/AC/ad/ad1/0 ==

== system rah/ac/Beaver dynamics/AC/ad/ad2/0 ==

== system rah/ac/Beaver dynamics/AC/ad/ad3/0 ==

== system rah/ac/Beaver dynamics/AC/ad/atm/0 ==

== system rah/ac/Beaver dynamics/AC/ae/aero/0 ==

== system rah/ac/Beaver dynamics/AC/ae/dl/0 ==

== system rah/ac/Beaver dynamics/AC/ae/fmdims/0 ==

== system rah/ac/Beaver dynamics/AC/eng/eng/0 ==

== system rah/ac/Beaver dynamics/AC/eng/fmdims/0 ==

== system rah/ac/Beaver dynamics/AC/eng/pow/0 ==

== system rah/ac/Beaver dynamics/AC/eqm/ODE/0 ==

== system rah/ac/Beaver dynamics/AC/eqm/ODE/Eulerdot ==
  note: ueul=[x;Ftot;Mtot;yhlp]
  note: yeul=[psi dot; theta dot; phi dot]
  ueul : Inport  Port=1  PortWidth=-1  SampleTime=-1
  0 : Subsystem
      settings: OpenFcn=fdchelp eulerdot
      mask Display: disp('EULERDOT\nM.O. Rauw, October 1997')
  Mux1 : Mux  Inputs=[29 1]
  Mux2 : Mux  Inputs=3
  phi dot : Fcn  Expr=u[4] + u[30]*u[26]
  psi dot : Fcn  Expr=(u[5]*u[28] + u[6]*u[29])/u[27]
  theta dot : Fcn  Expr=u[5]*u[29] - u[6]*u[28]
  yeul : Outport  Port=1  InitialOutput=0
  wires:
  ueul/1 -> theta dot/1, Mux1/1, psi dot/1
  psi dot/1 -> Mux2/1, Mux1/2
  theta dot/1 -> Mux2/2
  Mux2/1 -> yeul/1
  phi dot/1 -> Mux2/3
  Mux1/1 -> phi dot/1

== system rah/ac/Beaver dynamics/AC/eqm/ODE/Vabdot ==
  note: yVab=[V dot;alpha dot;beta dot]
  note: uVab=[x;Ftot;Mtot;yhlp]
  uVab : Inport  Port=1  PortWidth=-1  SampleTime=-1
  0 : Subsystem
      settings: OpenFcn=fdchelp vabdot
      mask Display: disp('VABDOT\nM.O. Rauw, October 1997')
  Mux2 : Mux  Inputs=3
  V dot : Fcn  Expr=(u[13]*u[19]*u[21]+u[14]*u[22]+u[15]*u[20]*u[21])/m
  alpha dot : Fcn  Expr=(-u[13]*u[20]+u[15]*u[19])/(m*u[1]*u[21]) - u[23]*(u[4]*u[19]+u[6]*u[20]) + u[5]
  beta dot : Fcn  Expr=(-u[13]*u[19]*u[22]+u[14]*u[21]-u[15]*u[20]*u[22])/(m*u[1]) + u[4]*u[20] - u[6]*u[19]
  yVab : Outport  Port=1  InitialOutput=0
  wires:
  beta dot/1 -> Mux2/3
  V dot/1 -> Mux2/1
  alpha dot/1 -> Mux2/2
  uVab/1 -> alpha dot/1, beta dot/1, V dot/1
  Mux2/1 -> yVab/1

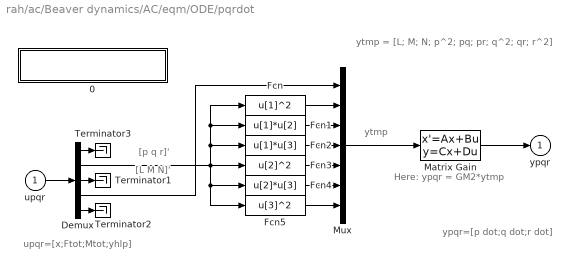
== system rah/ac/Beaver dynamics/AC/eqm/ODE/pqrdot ==
  note: ytmp = [L; M; N; p^2; pq; pr; q^2; qr; r^2]
  note: upqr=[x;Ftot;Mtot;yhlp]
  note: ypqr=[p dot;q dot;r dot]
  note: ytmp
  note: Here: ypqr = GM2*ytmp
  note: [L M N]'
  note: [p q r]'
  upqr : Inport  Port=1  PortWidth=-1  SampleTime=-1
  0 : Subsystem
      settings: OpenFcn=fdchelp pqrdot
      mask Display: disp('PQRDOT\nM.O. Rauw, October 1997')
  Demux : Demux  Outputs=[3 3 9 3 11]
  Fcn : Fcn  Expr=u[1]^2
  Fcn1 : Fcn  Expr=u[1]*u[2]
  Fcn2 : Fcn  Expr=u[1]*u[3]
  Fcn3 : Fcn  Expr=u[2]^2
  Fcn4 : Fcn  Expr=u[2]*u[3]
  Fcn5 : Fcn  Expr=u[3]^2
  Matrix Gain : StateSpace  A=A  B=B  C=C  D=D  X0=0  mask(Matrix Gain){@1=GM2}
      mask prompts: @1 "Gain matrix:"
      mask help: Matrix Gain
      mask init:
      | A = []; B = []; C = []; D = @1;
      mask Help: This block implements an matrix gain.\nThe matrix dimensions must be in accordance\nwith the dimension of the inputvector.
      mask Display: disp('y = A*u')
  Mux : Mux  Inputs=[3 1 1 1 1 1 1]
  Terminator1 : Terminator
  Terminator2 : Terminator
  Terminator3 : Terminator
  ypqr : Outport  Port=1  InitialOutput=0
  wires:
  Mux/1 -> Matrix Gain/1
  Matrix Gain/1 -> ypqr/1
  Fcn5/1 -> Mux/7
  Fcn4/1 -> Mux/6
  Fcn3/1 -> Mux/5
  Fcn2/1 -> Mux/4
  Fcn1/1 -> Mux/3
  Fcn/1 -> Mux/2
  Demux/4 -> Mux/1
  Demux/2 -> Fcn3/1, Fcn5/1, Fcn4/1, Fcn2/1, Fcn/1, Fcn1/1
  Demux/3 -> Terminator1/1
  Demux/5 -> Terminator2/1
  Demux/1 -> Terminator3/1
  upqr/1 -> Demux/1

== system rah/ac/Beaver dynamics/AC/eqm/ODE/xyHdot ==
  note: uxyH=[x;Ftot;Mtot;yhlp]
  note: yxyH=[xe dot; ye dot; H dot]
  ybvel* : Inport  Port=1  PortWidth=-1  SampleTime=-1
  uxYH : Inport  Port=2  PortWidth=-1  SampleTime=-1
  0 : Subsystem
      settings: OpenFcn=fdchelp xyhdot
      mask Display: disp('XYHDOT\nM.O. Rauw, October 1997')
  H dot : Fcn  Expr=u[30]*u[26] - (u[31]*u[28]+u[32]*u[29])*u[27]
  Mux2 : Mux  Inputs=[29 3]
  Mux3 : Mux  Inputs=2
  Mux4 : Mux  Inputs=[29 2]
  Mux5 : Mux  Inputs=3
  tmp1 : Fcn  Expr=u[30]*u[27] + (u[31]*u[28]+u[32]*u[29])*u[26]
  tmp2 : Fcn  Expr=u[31]*u[29] - u[32]*u[28]
  xe dot : Fcn  Expr=u[30]*u[25] - u[31]*u[24]
  ye dot : Fcn  Expr=u[30]*u[24] + u[31]*u[25]
  yxyH : Outport  Port=1  InitialOutput=0
  wires:
  uxYH/1 -> Mux2/1, Mux4/1
  ybvel*/1 -> Mux2/2
  Mux3/1 -> Mux4/2
  Mux2/1 -> tmp1/1, tmp2/1, H dot/1
  Mux4/1 -> xe dot/1, ye dot/1
  Mux5/1 -> yxyH/1
  ye dot/1 -> Mux5/2
  tmp2/1 -> Mux3/2
  xe dot/1 -> Mux5/1
  H dot/1 -> Mux5/3
  tmp1/1 -> Mux3/1

== system rah/ac/Beaver dynamics/AC/eqm/uvw/0 ==

== system rah/ac/Beaver dynamics/AC/eqm/xdotcorr/0 ==

== system rah/ac/Beaver dynamics/AC/out/accel/0 ==

== system rah/ac/Beaver dynamics/AC/out/fp/0 ==

== system rah/ac/Beaver dynamics/AC/out/uvwdot/0 ==

== system rah/ac/Beaver dynamics/AC/eqm/ODE/Eulerdot/0 ==

== system rah/ac/Beaver dynamics/AC/eqm/ODE/Vabdot/0 ==

== system rah/ac/Beaver dynamics/AC/eqm/ODE/pqrdot/0 ==

== system rah/ac/Beaver dynamics/AC/eqm/ODE/xyHdot/0 ==
